simulink model "gridconnectedpvarray"  (R2023b)
settings: Solver=FixedStepDiscrete  StartTime=0.0  StopTime=2.5  RelTol=1e-3
PreLoadFcn:
  | Ts_Power=1e-6;
  | Ts_Control=100e-6;
InitFcn:
  | Ts_Power=1e-6;
  | Ts_Control=100e-6;
undefined symbols (not defined in the file): D1, Delta, DiscIntNeverNeededParam
libraries: spsSeriesRLCBranchLib x5, spsMeanLib x3, spsThreePhaseTransformerTwoWindingsLib x2, spsDistributedParametersLineLib x2, spsThreePhaseParallelRLCLoadLib x2, spsFourierLib x2, slpidlib x2, spsabctodq0Lib x2, spsVoltageMeasurementLib x2, spsThreePhaseSeriesRLCLoadLib x1, spsThreeLevelBridgeLib x1, spsThreePhaseSourceLib x1
(part 1 of 2)
settings Model: SimulationMode=accelerator  Creator=The MathWorks, Inc.  LastModifiedBy=HP
settings SolverCC: AlgebraicLoopSolver=TrustRegion
settings DataIOCC: LimitDataPoints=on  SaveFormat=Array  SignalLogging=off  DSMLogging=off  ReturnWorkspaceOutputs=off
settings OptimizationCC: ExpressionDepthLimit=2147483647  EfficientMapNaN2IntZero=off  LifeSpan=inf
settings DebuggingCC: UnderspecifiedInitializationDetection=Classic  MergeDetectMultiDrivingBlocksExec=none  SolverPrmCheckMsg=warning  FcnCallInpInsideContextMsg=warning  UnconnectedInputMsg=warning  UnconnectedOutputMsg=warning  UnconnectedLineMsg=warning  StateNameClashWarn=warning  SubsystemReferenceDiagnosticForUnitTest=warning  SFUnexpectedBacktrackingDiag=warning  SFNoUnconditionalDefaultTransitionDiag=warning  SFExecutionAtInitializationDiag=none  ArithmeticOperatorsInVariantConditions=warning
settings HardwareCC: ProdBitPerPointer=32  ProdBitPerSizeT=32  ProdBitPerPtrDiffT=32  ProdLargestAtomicFloat=None  ProdIntDivRoundTo=Undefined  ProdEndianess=Unspecified  ProdWordSize=32  ProdHWDeviceType=32-bit Generic  TargetBitPerPointer=64  TargetBitPerSizeT=64  TargetBitPerPtrDiffT=64  TargetLongLongMode=on  TargetIntDivRoundTo=Zero  TargetEndianess=LittleEndian  TargetWordSize=64  TargetHWDeviceType=MATLAB Host  ProdEqTarget=off
settings ModelReferenceCC: EnableRefExpFcnMdlSchedulingChecks=on  PropagateSignalLabelsOutOfModel=off
settings SFSimCC: SimUseLocalCustomCode=off  CustomCodeUndefinedFunction=UseInterfaceOnly
settings CodeAppCC: MaxIdLength=128
settings GRTTargetCC: TargetLangStandard=C89/C90 (ANSI)  CombineOutputUpdateFcns=off  GRTInterface=on
settings ConfigComp: CovMetricSettings=dw  CovSaveCumulativeToWorkspaceVar=on  CovSaveSingleToWorkspaceVar=on  CovExternalEMLEnable=off  CovSFcnEnable=off
settings SimscapeCC: SimscapeNormalizeSystem=off

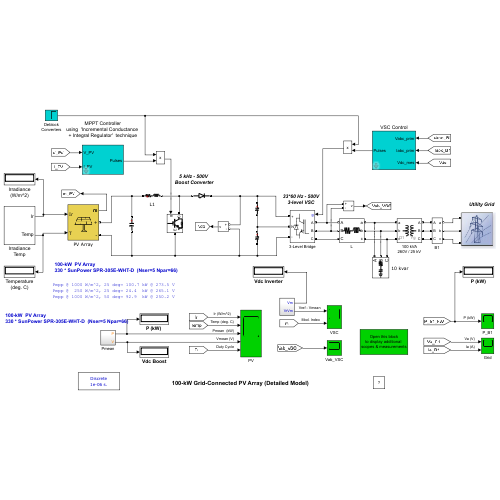
[thumbnail: Simulink's stored preview of the top-level diagram]
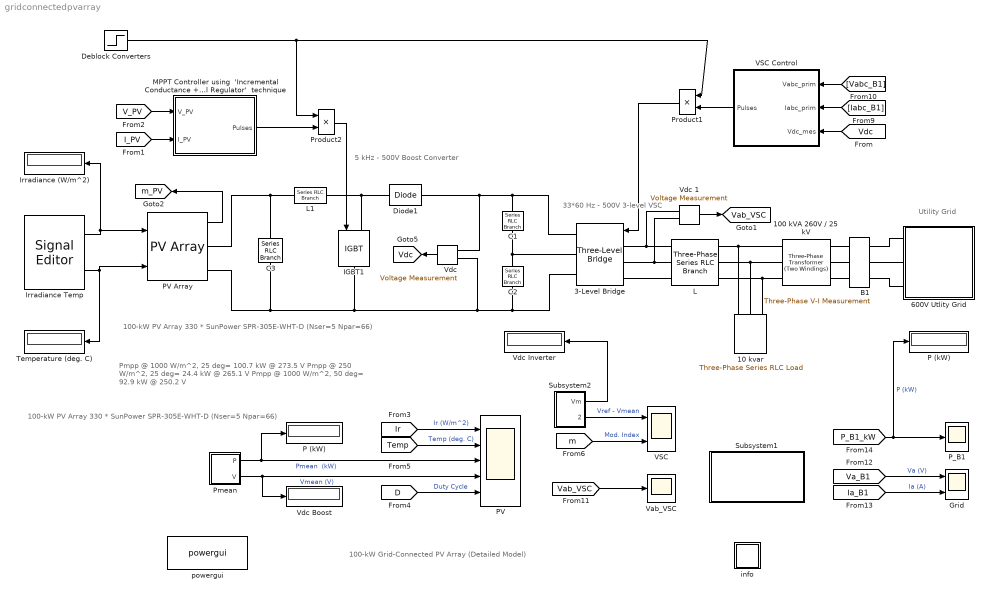
== system gridconnectedpvarray ==
  note: 5 kHz - 500V
      | Boost Converter
  note: 33*60 Hz - 500V
      | 3-level VSC
  note: 100-kW Grid-Connected PV Array (Detailed Model)
  note: Utility Grid
  note: Pmpp @ 1000 W/m^2, 25 deg= 100.7 kW @ 273.5 V
      | Pmpp @  250 W/m^2, 25 deg= 24.4  kW @ 265.1 V
      | Pmpp @ 1000 W/m^2, 50 deg= 92.9  kW @ 250.2 V
  note: 100-kW  PV Array
      | 330 * SunPower SPR-305E-WHT-D  (Nser=5 Npar=66)
  note: 100-kW  PV Array
      | 330 * SunPower SPR-305E-WHT-D  (Nser=5 Npar=66)
  10 kvar : spsThreePhaseSeriesRLCLoadLib/Three-Phase Series RLC Load  LConnTagsString=A|B|C  Configuration=Y (grounded)  NominalVoltage=240  Vabc=[1e3 1e3 1e3]  Vabcp=[1e3 1e3 1e3]  NominalFrequency=60  UnbalancedPower=off  ActivePower=10e3/100  InductivePower=0  CapacitivePower=10e3  Pabc=[10e3 9e3 11e3]  QLabc=[100 90 110]  QCabc=[100 90 110]  Pabcp=[10e3 9e3 11e3]  QLabcp=[100 90 110]  QCabcp=[100 90 110]  Measurements=None  LoadType=constant Z
  100 kVA 260V / 25 kV : spsThreePhaseTransformerTwoWindingsLib/Three-Phase Transformer (Two Windings)  Winding1Connection=Yg  Winding2Connection=Delta (D1)  CoreType=Three single-phase transformers  SetSaturation=off  Hysteresis=off  DataFile='hysteresis'  SetInitialFlux=off  Measurements=None  UNITS=pu  NominalPower=[100e3 , 60 ]  Winding1=[ 25e3 , 0.001 , 0.03 ]  Winding2=[ 260 , 0.001 , 0.03 ]  Rm=500  Lm=500  L0=0.5  Saturation=[ 0,0 ; 0.0024,1.2 ; 1.0,1.52 ]  InitialFluxes=[ 0.8 , -0.8 , 0.7 ]  BreakLoop=off  DiscreteSolver=Trapezoidal iterative  DataType=off  TransfoNumber=0
  3-Level Bridge : spsThreeLevelBridgeLib/Three-Level Bridge  Arms=3  SnubberResistance=1e6  SbubberCapacitance=inf  Device=IGBT / Diodes  Ron=0.2e-3  ForwardVoltages="[  0  0 ]"  Measurements=None
      settings: AttributesFormatString=\n
  600V Utlity Grid : Subsystem
      mask Display: image('$imagefile')
  B1 : spsThreePhaseVIMeasurementLib/Three-Phase V-I Measurement  VoltageMeasurement=phase-to-ground  SetLabelV=on  LabelV=Vabc_B1  Vpu=off  VpuLL=off  CurrentMeasurement=yes  SetLabelI=on  LabelI=Iabc_B1  Ipu=off  Pbase=100e6  Vbase=500e3  OutputType=Magnitude  PhasorSimulation=off  PSBequivalent=0
  C1 : spsSeriesRLCBranchLib/Series RLC Branch  LConnTagsString=__new0  RConnTagsString=__new0  BranchType=C  Resistance=1.0  Inductance=1.0  SetiL0=off  InitialCurrent=0  Capacitance=12000e-06  Setx0=off  InitialVoltage=0  Measurements=None
  C2 : spsSeriesRLCBranchLib/Series RLC Branch  LConnTagsString=__new0  RConnTagsString=__new0  BranchType=C  Resistance=1.0  Inductance=1.0  SetiL0=off  InitialCurrent=0  Capacitance=12000e-06  Setx0=off  InitialVoltage=0  Measurements=None
  C3 : spsSeriesRLCBranchLib/Series RLC Branch  LConnTagsString=__new0  RConnTagsString=__new0  BranchType=C  Resistance=1.0  Inductance=1.0  SetiL0=off  InitialCurrent=0  Capacitance=100e-6  Setx0=off  InitialVoltage=0  Measurements=Branch voltage
  Deblock Converters : Step  Time=0.05  SampleTime=0
  Diode1 : spsDiodeLib/Diode  Ron=1e-4  Lon=0  Vf=0  IC=0  UseSnubber=off  Rs=inf  Cs=inf  Measurements=off
  Grid : Scope  NumInputPorts=2
  IGBT1 : spsIGBTLib/IGBT  Ron=0.001  Lon=0  Vf=0  Tf=0  Tt=0  IC=0  Rs=1e5  Cs=inf  Measurements=off
  Irradiance (W/m^2) : Display
      settings: Format=bank  Decimation=1000
  Irradiance Temp : SignalEditorBlockLib/Signal Editor  FileName=PVArrayGridData.mat  ActiveScenario=Ramp_up_down_Irradiance  ActiveSignal=Temp  IsBus=off  OutputBusObjectStr=Bus: BusObject  SampleTime=0  OutputAfterFinalValue=Extrapolation  Unit=inherit  PreserveSignalName=on  ApplySigPropsToAllScenarios=on  ApplySigPropsToAllSignals=off
  L : spsThreePhaseSeriesRLCBranchLib/Three-Phase Series RLC Branch  LConnTagsString=A|B|C  RConnTagsString=A|B|C  BranchType=RL  Resistance=500e-6*377/50/2  Inductance=500e-6/2  Capacitance=inf  Measurements=None
  L1 : spsSeriesRLCBranchLib/Series RLC Branch  LConnTagsString=__new0  RConnTagsString=__new0  BranchType=RL  Resistance=0.005  Inductance=5e-3  SetiL0=off  InitialCurrent=0  Capacitance=1e-6  Setx0=off  InitialVoltage=0  Measurements=None
  "MPPT Controller using  'Incremental Conductance + Integral Regulator'  technique " : Subsystem  mask(Boost Control - MPPT){fc=5000, T_MPPT=200e-6, Dinit=0.5}
      mask prompts: fc "PWM switching frequency (Hz)"; T_MPPT "Time window used by MPPT control (s)"; Dinit "Initial value of duty cycle"
  P (kW) : Display
      settings: Format=bank  Decimation=2000
  "P (kW) " : Display
      settings: Format=bank  Decimation=2000
  PV : Scope  NumInputPorts=5
  PV Array : spsPVArrayLib/PV Array  Npar=66  Nser=5  PlotType=array @ 1000 W/m2 & specified temperatures  S_vec="[ 1000  250 ]"  Temp_C_vec="[0 25 50  ]"  ModuleName=SunPower SPR-305E-WHT-D  PlotWhenSelected=off  Pm=305.226  Ncell=96  Voc=64.2  Isc=5.96  Vm=54.7  Im=5.58  beta_Voc_pc=-0.2727  alpha_Isc_pc=0.061745  beta_Voc=-0.17507  alpha_Isc=0.00368  IL=5.9657  I0=6.3076e-12  nI=0.94489  Rsh=393.2054  Rs=0.37428  RobustModel=off  RobustCellTemperature=25  BAL=on  Tc=1e-6  Tfilter=5e-5
  P_B1 : Scope
  Pmean : Subsystem
  Product1 : Product  RndMeth=Zero
  Product2 : Product  RndMeth=Zero
  Subsystem1 : Subsystem
      mask Display: disp('Open this block\nto display additional \nscopes & measurements')
  Subsystem2 : Subsystem
  Temperature (deg. C) : Display
      settings: Format=bank  Decimation=1000
  VSC : Scope  NumInputPorts=2
  VSC Control : Subsystem  mask(VSC Main Controller){nom=[ 100e3  60 ], Vnom=[ 25e3 260 ], Vnom_dc=500, RLxfo=[0.002  0.06 ], RLchoke=[2e-3  250e-6  ], K_VDCreg=[7  800], K_Ireg=[0.3 20], Ts=Ts_Control}
      mask prompts: nom "Nominal power and frequency [ Pnom(VA)  Fnom(Hz) ]:"; Vnom "Nominal primary and secondary voltages (Vrms LL) [ Vnom_prim   Vnom_sec ]:"; Vnom_dc "Nominal DC bus voltage (V):"; RLxfo "Total transformer leakage impedance (pu/Pnom) [ Rxfo  Lxf ]"; RLchoke "Choke impedance [ R(ohm) L(H) ]"; K_VDCreg "VDC regultator gains [ Kp  Ki ]:"; K_Ireg "Current regulator gains [ Kp  Ki ]:"; Ts "Sample time"
      mask init:
      | Pnom=nom(1);
      | Fnom=nom(2);
      | Vnom_prim=Vnom(1);
      | Vnom_sec=Vnom(2);
      | Zbase=Vnom_sec^2/Pnom;
      | Rtot_pu=RLxfo(1) + RLchoke(1)/Zbase;
      | Ltot_pu=RLxfo(2) + RLchoke(2)/(Zbase/(2*pi*Fnom));
      | Kp_VDCreg=K_VDCreg(1);
      | Ki_VDCreg=K_VDCreg(2);
      | Kp_Ireg=K_Ireg(1);
      | Ki_Ireg=K_Ireg(2);
      | Vdc_ref=Vnom_dc;
      | % Used to determine initial value of Boost Control (MPPT)
      | assignin('base','Vdc_ref_Inv',Vdc_ref);
  Vab_VSC : Scope
  "Vdc " : spsVoltageMeasurementLib/Voltage Measurement  Tag=PoWeRsYsTeMmEaSuReMeNt  PhasorSimulation=off  OutputType=Magnitude  PSBequivalent=0
  Vdc 1 : spsVoltageMeasurementLib/Voltage Measurement  Tag=PoWeRsYsTeMmEaSuReMeNt  PhasorSimulation=off  OutputType=Magnitude  PSBequivalent=0
  Vdc Boost : Display
      settings: Format=bank  Decimation=2000
  Vdc Inverter : Display
      settings: Format=bank  Decimation=2000
  info : Subsystem
      settings: OpenFcn="showExample(\"simscapeelectricalsps/PVArrayGridExample\")"
      mask Display: disp('?')
  powergui : spspowerguiLib/powergui  Priority=1  SimulationMode=Discrete  SampleTime=Ts_Power  frequency=60  Iterations=50  frequencyindice=0  Pbase=100e6  ErrMax=1e-4  UnitsV=kV  UnitsW=MW  buscounter=0  FunctionMessages=off  echomessages=off  EnableUseOfTLC=off  CurrentSourceSwitches=off  DisableSnubberDevices=off  DisableRonSwitches=off  DisableVfSwitches=off  DisplayEquations=off  AutomaticDiscreteSolvers=off  SolverType=Tustin/Backward Euler (TBE)  Interpol=off  ExternalGateDelay=off  methode=off  Ts=0  x0status=blocks  SPID=off  SwTol=0  HookPort=off  NonlinearTolerance=1e-8  nMaxIteration=10  ContinueOnMaxIteration=off  RestoreLinks=warning  ResistiveCurrentMeasurement=off  Frange=[0:2:500]  Ylog=off  Xlog=on  ShowGrid=off  save=off  variable=ZData  structure=0  ZoomFFT=on  StartTime=0.0  cycles=1  DisplayStyle=1  fundamental=60  FreqAxis=off  MaxFrequency=1000  frequencyindicesteady=1  RmsSteady=1  display=off
  tag scope: Vab_VSC=global, Vdc=global, m_PV=global
  wires:
  "Vdc "/1 -> [Vdc]
  Product2/1 -> IGBT1/1
  "MPPT Controller using  'Incremental Conductance + Integral Regulator'  technique "/1(Pulses) -> Product2/2
  Deblock Converters/1 -> Product1/1, Product2/1
  [Vabc_B1] -> VSC Control/1(Vabc_prim)
  [Iabc_B1] -> VSC Control/2(Iabc_prim)
  [Vdc] -> VSC Control/3(Vdc_mes)
  VSC Control/1(Pulses) -> Product1/2
  Product1/1 -> 3-Level Bridge/1
  [I_PV] -> "MPPT Controller using  'Incremental Conductance + Integral Regulator'  technique "/2(I_PV)
  [V_PV] -> "MPPT Controller using  'Incremental Conductance + Integral Regulator'  technique "/1(V_PV)
  Pmean/1(P) -> "P (kW) "/1, PV/3  "Pmean  (kW)"
  [m] -> VSC/2  "Mod. Index"
  Vdc 1/1 -> [Vab_VSC]
  [Vab_VSC] -> Vab_VSC/1
  [Ia_B1] -> Grid/2  "Ia (A)"
  [Va_B1] -> Grid/1  "Va (V)"
  [P_B1_kW] -> P_B1/1, P (kW)/1  "P (kW)"
  Pmean/2(V) -> Vdc Boost/1, PV/4  "Vmean (V)"
  Subsystem2/2(VrVm) -> VSC/1  "Vref - Vmean"
  Subsystem2/1(Vm) -> Vdc Inverter/1
  PV Array/1 -> [m_PV]
  Irradiance Temp/1 -> PV Array/1, Irradiance (W/m^2)/1
  Irradiance Temp/2 -> PV Array/2, Temperature (deg. C)/1
  [D] -> PV/5  "Duty Cycle"
  [Temp] -> PV/2  "Temp (deg. C)"
  [Ir] -> PV/1  "Ir (W/m^2)"
  connections:
  3-Level Bridge/RConn1 -- Diode1/RConn1 -- "Vdc "/LConn1 -- C1/LConn1
  L1/RConn1 -- Diode1/LConn1 -- IGBT1/LConn1
  3-Level Bridge/RConn3 -- C2/RConn1 -- "Vdc "/LConn2 -- IGBT1/RConn1 -- PV Array/RConn2 -- C3/RConn1
  3-Level Bridge/LConn1 -- L/LConn1 -- Vdc 1/LConn1
  3-Level Bridge/LConn2 -- L/LConn2 -- Vdc 1/LConn2
  3-Level Bridge/LConn3 -- L/LConn3
  L/RConn1 -- 100 kVA 260V / 25 kV/RConn1 -- 10 kvar/LConn1
  L/RConn2 -- 100 kVA 260V / 25 kV/RConn2 -- 10 kvar/LConn2
  L/RConn3 -- 100 kVA 260V / 25 kV/RConn3 -- 10 kvar/LConn3
  B1/LConn1 -- 100 kVA 260V / 25 kV/LConn1
  B1/LConn2 -- 100 kVA 260V / 25 kV/LConn2
  B1/LConn3 -- 100 kVA 260V / 25 kV/LConn3
  C2/LConn1 -- C1/RConn1 -- 3-Level Bridge/RConn2
  C3/LConn1 -- PV Array/RConn1 -- L1/LConn1
  B1/RConn2 -- 600V Utlity Grid/LConn2
  B1/RConn1 -- 600V Utlity Grid/LConn1
  B1/RConn3 -- 600V Utlity Grid/LConn3

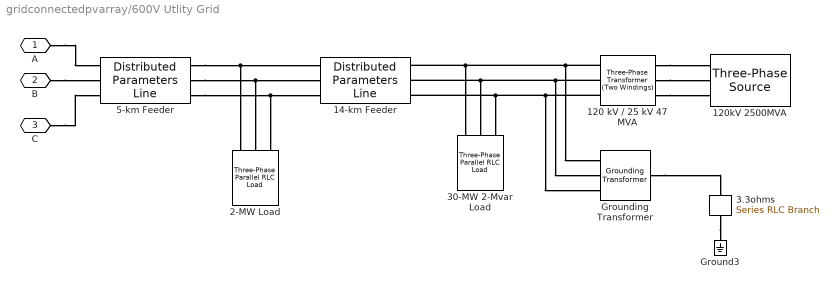
== system gridconnectedpvarray/600V Utlity Grid ==
  120 kV / 25 kV 47 MVA : spsThreePhaseTransformerTwoWindingsLib/Three-Phase Transformer (Two Windings)  Winding1Connection=Yg  Winding2Connection=Delta (D1)  CoreType=Three single-phase transformers  SetSaturation=off  Hysteresis=off  DataFile='basic_model'  SetInitialFlux=off  Measurements=None  UNITS=pu  NominalPower=[47e6 60 ]  Winding1="[ 120e3  0.08/30   0.08 ]"  Winding2="[ 25e3  0.08/30  0.08]"  Rm=500  Lm=500  L0=0.5  Saturation="[ 0,0  ;  0.005,1.2  ;  1.0,1.4 ]"  InitialFluxes=[ 0.8 , -0.8 , 0.7 ]  BreakLoop=off  DiscreteSolver=Trapezoidal iterative  DataType=off  TransfoNumber=0
  120kV 2500MVA : spsThreePhaseSourceLib/Three-Phase Source  InternalConnection=Yg  VoltagePhases=off  Voltage=120e3  PhaseAngle=0  Voltage_phases=[25e3 25e3 25e3]/sqrt(3)  PhaseAngles_phases=[0 -120 +120]  Frequency=60  NonIdealSource=on  SpecifyImpedance=on  Resistance=0.8929  Inductance=16.58e-3  ShortCircuitLevel=2500e6  BaseVoltage=120e3  XRratio=7  BusType=swing  Pref=0  Qref=0  Prefabc=[10e3, 10e3, 10e3]  Qrefabc=[0, 0, 0]  Qmin=-inf  Qmax=inf
  14-km Feeder : spsDistributedParametersLineLib/Distributed Parameters Line  Phases=3  Length=14  Frequency=60  Resistance=[0.1153 0.413]  Inductance=[1.05e-3 3.32e-3]  Capacitance=[11.33e-009 5.01e-009]  x1=[-5.8e-05 6.66844526107812e-10 0 0;-5.7e-05 6.67988838949903e-10 0 0;-5.6e-05 6.69133056855883e-10 0 0;-5.5e-05 6.70277179663133e-10 0 0;-5.4e-05 6.71421207209047e-10 0 0;-5.3e-05 6.72565139331033e-10 0 0;-5.2e-05 6.73708975866514e-10 0 0;-5.1e-05 6.74852716652925e-10 0 0;-5e-05 6.75996361527714e-10 0 0;-4.9e-05 6.77139910328345e-10 -3790.73535190058 -24061.4134200257;-4.8e-05 6.78283362892292e-10 -3781.66414358518 -24062.8407837201;-4.7e-05 6.79426719057047e-10 -3772.59239781097 -24064.2647275482;-4.6e-05 6.80569978660113e-10 -3763.52011586725 -24065.6852513076;-4.5e-05 6.81713141539008e-10 -3754.44729904339 -24067.1023547964;-4.4e-05 6.82856207531261e-10 -3745.37394862884 -24068.5160378133;-4.3e-05 6.83999176474418e-10 -3736.30006591311 -24069.9263001572;-4.2e-05 6.85142048206038e-10 -3727.22565218583 -24071.3331416278;-4.1e-05 6.86284822563693e-10 -3718.15070873665 -24072.7365620252;-4e-05 6.8742749938497e-10 -3709.07523685534 -24074.1365611498;-3.9e-05 6.88570078507468e-10 -3699.99923783172 -24075.5331388027;-3.8e-05 6.89712559768802e-10 -3690.92271295569 -24076.9262947854;-3.7e-05 6.90854943006599e-10 -3681.84566351723 -24078.3160289;-3.6e-05 6.91997228058502e-10 -3672.76809080639 -24079.7023409488;-3.5e-05 6.93139414762165e-10 -3663.6899961133 -24081.0852307349;-3.4e-05 6.9428150295526e-10 -3654.61138072814 -24082.4646980618;-3.3e-05 6.9542349247547e-10 -3645.53224594121 -24083.8407427334;-3.2e-05 6.96565383160492e-10 -3636.45259304285 -24085.213364554;-3.1e-05 6.97707174848038e-10 -3627.37242332347 -24086.5825633288;-3e-05 6.98848867375835e-10 -3618.29173807357 -24087.9483388629;-2.9e-05 6.99990460581623e-10 -3609.21053858373 -24089.3106909624;-2.8e-05 7.01131954303155e-10 -3600.12882614457 -24090.6696194337;-2.7e-05 7.022733483782e-10 -3591.04660204683 -24092.0251240835;-2.6e-05 7.0341464264454e-10 -3581.96386758127 -24093.3772047192;-2.5e-05 7.04555836939972e-10 -3572.88062403876 -24094.7258611487;-2.4e-05 7.05696931102307e-10 -3563.79687271023 -24096.0710931803;-2.3e-05 7.0683792496937e-10 -3554.71261488669 -24097.4129006229;-2.2e-05 7.07978818378999e-10 -3545.62785185921 -24098.7512832856;-2.1e-05 7.0911961116905e-10 -3536.54258491894 -24100.0862409784;-2e-05 7.1026030317739e-10 -3527.4568153571 -24101.4177735114;-1.9e-05 7.114008942419e-10 -3518.37054446498 -24102.7458806954;-1.8e-05 7.12541384200478e-10 -3509.28377353393 -24104.0705623418;-1.7e-05 7.13681772891034e-10 -3500.1965038554 -24105.3918182621;-1.6e-05 7.14822060151494e-10 -3491.10873672089 -24106.7096482687;-1.5e-05 7.15962245819797e-10 -3482.02047342196 -24108.0240521742;-1.4e-05 7.17102329733899e-10 -3472.93171525028 -24109.3350297919;-1.3e-05 7.18242311731766e-10 -3463.84246349754 -24110.6425809353;-1.2e-05 7.19382191651383e-10 -3454.75271945554 -24111.9467054188;-1.1e-05 7.20521969330747e-10 -3445.66248441613 -24113.2474030568;-1e-05 7.21661644607871e-10 -3436.57175967124 -24114.5446736647;-9e-06 7.2280121732078e-10 -3427.48054651286 -24115.838517058;-8e-06 7.23940687307517e-10 -3418.38884623305 -24117.1289330527;-7e-06 7.25080054406137e-10 -3409.29666012396 -24118.4159214656;-6e-06 7.26219318454711e-10 -3400.20398947777 -24119.6994821138;-5e-06 7.27358479291324e-10 -3391.11083558677 -24120.9796148147;-4e-06 7.28497536754075e-10 -3382.01719974329 -24122.2563193865;-3e-06 7.2963649068108e-10 -3372.92308323975 -24123.5295956477;-2e-06 7.30775340910467e-10 -3363.82848736861 -24124.7994434173;-1e-06 7.31914087280381e-10 -3354.73341342242 -24126.0658625149]  x2=[-5.8e-05 8.33047014327362e-10 0 0;-5.7e-05 8.34243099749187e-10 0 0;-5.6e-05 8.35439066606464e-10 0 0;-5.5e-05 8.36634914729217e-10 0 0;-5.4e-05 8.37830643947491e-10 0 0;-5.3e-05 8.39026254091345e-10 0 0;-5.2e-05 8.40221744990856e-10 0 0;-5.1e-05 8.4141711647612e-10 0 0;-5e-05 8.42612368377246e-10 0 0;-4.9e-05 8.43807500524362e-10 -3379.3924259141 -24244.0512732158;-4.8e-05 8.45002512747615e-10 -3370.2523939823 -24245.3235513057;-4.7e-05 8.46197404877165e-10 -3361.11188306246 -24246.5923835944;-4.6e-05 8.47392176743193e-10 -3351.97089445368 -24247.8577699016;-4.5e-05 8.48586828175894e-10 -3342.82942945507 -24249.1197100474;-4.4e-05 8.49781359005482e-10 -3333.68748936585 -24250.3782038526;-4.3e-05 8.50975769062187e-10 -3324.54507548529 -24251.6332511381;-4.2e-05 8.52170058176258e-10 -3315.40218911273 -24252.8848517258;-4.1e-05 8.53364226177958e-10 -3306.25883154759 -24254.1330054376;-4e-05 8.5455827289757e-10 -3297.11500408932 -24255.3777120962;-3.9e-05 8.55752198165393e-10 -3287.97070803749 -24256.6189715247;-3.8e-05 8.56946001811744e-10 -3278.82594469169 -24257.8567835466;-3.7e-05 8.58139683666958e-10 -3269.6807153516 -24259.0911479861;-3.6e-05 8.59333243561384e-10 -3260.53502131696 -24260.3220646678;-3.5e-05 8.60526681325391e-10 -3251.38886388758 -24261.5495334167;-3.4e-05 8.61719996789366e-10 -3242.24224436333 -24262.7735540582;-3.3e-05 8.62913189783712e-10 -3233.09516404414 -24263.9941264186;-3.2e-05 8.64106260138849e-10 -3223.94762423004 -24265.2112503243;-3.1e-05 8.65299207685215e-10 -3214.79962622107 -24266.4249256023;-3e-05 8.66492032253267e-10 -3205.65117131739 -24267.6351520801;-2.9e-05 8.67684733673476e-10 -3196.50226081918 -24268.8419295858;-2.8e-05 8.68877311776334e-10 -3187.35289602671 -24270.0452579477;-2.7e-05 8.70069766392348e-10 -3178.20307824031 -24271.245136995;-2.6e-05 8.71262097352045e-10 -3169.05280876038 -24272.4415665571;-2.5e-05 8.72454304485967e-10 -3159.90208888736 -24273.6345464639;-2.4e-05 8.73646387624675e-10 -3150.75091992179 -24274.8240765459;-2.3e-05 8.74838346598747e-10 -3141.59930316424 -24276.010156634;-2.2e-05 8.7603018123878e-10 -3132.44723991538 -24277.1927865597;-2.1e-05 8.77221891375388e-10 -3123.29473147589 -24278.3719661549;-2e-05 8.78413476839201e-10 -3114.14177914658 -24279.547695252;-1.9e-05 8.79604937460869e-10 -3104.98838422826 -24280.7199736838;-1.8e-05 8.80796273071058e-10 -3095.83454802185 -24281.8888012839;-1.7e-05 8.81987483500454e-10 -3086.68027182831 -24283.054177886;-1.6e-05 8.83178568579759e-10 -3077.52555694867 -24284.2161033246;-1.5e-05 8.84369528139693e-10 -3068.370404684 -24285.3745774345;-1.4e-05 8.85560362010994e-10 -3059.21481633548 -24286.529600051;-1.3e-05 8.86751070024418e-10 -3050.0587932043 -24287.6811710101;-1.2e-05 8.87941652010739e-10 -3040.90233659175 -24288.829290148;-1.1e-05 8.89132107800748e-10 -3031.74544779915 -24289.9739573016;-1e-05 8.90322437225256e-10 -3022.58812812792 -24291.1151723082;-9e-06 8.9151264011509e-10 -3013.4303788795 -24292.2529350056;-8e-06 8.92702716301095e-10 -3004.27220135543 -24293.3872452321;-7e-06 8.93892665614136e-10 -2995.11359685727 -24294.5181028264;-6e-06 8.95082487885093e-10 -2985.95456668667 -24295.645507628;-5e-06 8.96272182944868e-10 -2976.79511214534 -24296.7694594765;-4e-06 8.97461750624376e-10 -2967.63523453504 -24297.8899582121;-3e-06 8.98651190754555e-10 -2958.47493515758 -24299.0070036758;-2e-06 8.99840503166358e-10 -2949.31421531486 -24300.1205957086;-1e-06 9.01029687690758e-10 -2940.15307630881 -24301.2307341524]  x3=[-5.8e-05 -3.7534649390882e-12 0 0;-5.7e-05 -3.74760398121956e-12 0 0;-5.6e-05 -3.74174249073282e-12 0 0;-5.5e-05 -3.73588046846102e-12 0 0;-5.4e-05 -3.7300179152373e-12 0 0;-5.3e-05 -3.72415483189484e-12 0 0;-5.2e-05 -3.71829121926693e-12 0 0;-5.1e-05 -3.7124270781869e-12 0 0;-5e-05 -3.7065624094882e-12 0 0;-4.9e-05 -3.70069721400432e-12 -23.5442847382658 -155.68147777383;-4.8e-05 -3.69483149256883e-12 -23.4855925321471 -155.690342696951;-4.7e-05 -3.68896524601538e-12 -23.426896988202 -155.699185493002;-4.6e-05 -3.68309847517771e-12 -23.3681981147723 -155.708006160726;-4.5e-05 -3.6772311808896e-12 -23.3094959202006 -155.716804698871;-4.4e-05 -3.67136336398493e-12 -23.2507904128296 -155.725581106184;-4.3e-05 -3.66549502529765e-12 -23.1920816010027 -155.73433538142;-4.2e-05 -3.65962616566178e-12 -23.1333694930639 -155.743067523333;-4.1e-05 -3.65375678591142e-12 -23.0746540973573 -155.751777530683;-4e-05 -3.64788688688073e-12 -23.0159354222278 -155.760465402232;-3.9e-05 -3.64201646940396e-12 -22.9572134760206 -155.769131136745;-3.8e-05 -3.63614553431543e-12 -22.8984882670813 -155.777774732991;-3.7e-05 -3.63027408244952e-12 -22.8397598037562 -155.78639618974;-3.6e-05 -3.62440211464071e-12 -22.7810280943919 -155.794995505769;-3.5e-05 -3.61852963172352e-12 -22.7222931473354 -155.803572679854;-3.4e-05 -3.61265663453258e-12 -22.6635549709343 -155.812127710777;-3.3e-05 -3.60678312390256e-12 -22.6048135735366 -155.820660597322;-3.2e-05 -3.60090910066822e-12 -22.5460689634907 -155.829171338275;-3.1e-05 -3.59503456566439e-12 -22.4873211491457 -155.837659932428;-3e-05 -3.58915951972597e-12 -22.4285701388508 -155.846126378575;-2.9e-05 -3.58328396368794e-12 -22.3698159409559 -155.854570675511;-2.8e-05 -3.57740789838535e-12 -22.3110585638113 -155.862992822037;-2.7e-05 -3.57153132465331e-12 -22.2522980157677 -155.871392816955;-2.6e-05 -3.56565424332702e-12 -22.1935343051762 -155.879770659072;-2.5e-05 -3.55977665524175e-12 -22.1347674403886 -155.888126347198;-2.4e-05 -3.55389856123282e-12 -22.0759974297569 -155.896459880144;-2.3e-05 -3.54801996213564e-12 -22.0172242816336 -155.904771256727;-2.2e-05 -3.5421408587857e-12 -21.9584480043718 -155.913060475764;-2.1e-05 -3.53626125201856e-12 -21.8996686063247 -155.921327536079;-2e-05 -3.53038114266982e-12 -21.8408860958464 -155.929572436495;-1.9e-05 -3.52450053157519e-12 -21.782100481291 -155.937795175842;-1.8e-05 -3.51861941957043e-12 -21.7233117710134 -155.945995752951;-1.7e-05 -3.51273780749138e-12 -21.6645199733688 -155.954174166655;-1.6e-05 -3.50685569617395e-12 -21.6057250967126 -155.962330415794;-1.5e-05 -3.50097308645411e-12 -21.5469271494011 -155.970464499207;-1.4e-05 -3.49508997916792e-12 -21.4881261397908 -155.978576415739;-1.3e-05 -3.4892063751515e-12 -21.4293220762384 -155.986666164236;-1.2e-05 -3.48332227524104e-12 -21.3705149671015 -155.994733743549;-1.1e-05 -3.4774376802728e-12 -21.3117048207378 -156.002779152532;-1e-05 -3.47155259108311e-12 -21.2528916455056 -156.010802390041;-9e-06 -3.46566700850838e-12 -21.1940754497635 -156.018803454935;-8e-06 -3.45978093338507e-12 -21.1352562418706 -156.026782346078;-7e-06 -3.45389436654974e-12 -21.0764340301865 -156.034739062336;-6e-06 -3.44800730883899e-12 -21.017608823071 -156.042673602577;-5e-06 -3.4421197610895e-12 -20.9587806288846 -156.050585965674;-4e-06 -3.43623172413803e-12 -20.8999494559881 -156.058476150503;-3e-06 -3.4303431988214e-12 -20.8411153127426 -156.066344155942;-2e-06 -3.42445418597649e-12 -20.7822782075098 -156.074189980873;-1e-06 -3.41856468644028e-12 -20.7234381486519 -156.082013624181]  x4=[-5.8e-05 5.86381987524126e-12 0 0;-5.7e-05 5.86113014706762e-12 0 0;-5.6e-05 5.85843958589666e-12 0 0;-5.5e-05 5.85574819211079e-12 0 0;-5.4e-05 5.8530559660925e-12 0 0;-5.3e-05 5.85036290822443e-12 0 0;-5.2e-05 5.84766901888932e-12 0 0;-5.1e-05 5.84497429847002e-12 0 0;-5e-05 5.84227874734953e-12 0 0;-4.9e-05 5.83958236591093e-12 -1.35581366009685 -2.15298522697963;-4.8e-05 5.83688515453745e-12 -1.35500190746171 -2.15349620368202;-4.7e-05 5.83418711361241e-12 -1.35418996225058 -2.15400687432457;-4.6e-05 5.83148824351927e-12 -1.35337782457886 -2.15451723883471;-4.5e-05 5.8287885446416e-12 -1.35256549456196 -2.1550272971399;-4.4e-05 5.82608801736309e-12 -1.35175297231535 -2.15553704916764;-4.3e-05 5.82338666206754e-12 -1.35094025795449 -2.15604649484551;-4.2e-05 5.82068447913887e-12 -1.35012735159489 -2.15655563410108;-4.1e-05 5.81798146896113e-12 -1.34931425335208 -2.157064466862;-4e-05 5.81527763191847e-12 -1.34850096334163 -2.15757299305595;-3.9e-05 5.81257296839516e-12 -1.34768748167912 -2.15808121261067;-3.8e-05 5.80986747877561e-12 -1.34687380848016 -2.15858912545391;-3.7e-05 5.80716116344432e-12 -1.34605994386039 -2.1590967315135;-3.6e-05 5.80445402278592e-12 -1.34524588793549 -2.1596040307173;-3.5e-05 5.80174605718515e-12 -1.34443164082114 -2.16011102299319;-3.4e-05 5.79903726702688e-12 -1.34361720263308 -2.16061770826914;-3.3e-05 5.79632765269608e-12 -1.34280257348704 -2.16112408647313;-3.2e-05 5.79361721457786e-12 -1.34198775349882 -2.16163015753318;-3.1e-05 5.79090595305742e-12 -1.3411727427842 -2.16213592137738;-3e-05 5.7881938685201e-12 -1.34035754145903 -2.16264137793385;-2.9e-05 5.78548096135135e-12 -1.33954214963916 -2.16314652713075;-2.8e-05 5.78276723193672e-12 -1.33872656744047 -2.16365136889629;-2.7e-05 5.78005268066191e-12 -1.33791079497889 -2.16415590315871;-2.6e-05 5.7773373079127e-12 -1.33709483237034 -2.16466012984631;-2.5e-05 5.77462111407503e-12 -1.3362786797308 -2.16516404888744;-2.4e-05 5.7719040995349e-12 -1.33546233717626 -2.16566766021046;-2.3e-05 5.76918626467848e-12 -1.33464580482273 -2.16617096374382;-2.2e-05 5.76646760989203e-12 -1.33382908278627 -2.16667395941597;-2.1e-05 5.76374813556193e-12 -1.33301217118295 -2.16717664715543;-2e-05 5.76102784207467e-12 -1.33219507012888 -2.16767902689076;-1.9e-05 5.75830672981688e-12 -1.33137777974017 -2.16818109855055;-1.8e-05 5.75558479917529e-12 -1.33056030013299 -2.16868286206346;-1.7e-05 5.75286205053673e-12 -1.32974263142352 -2.16918431735816;-1.6e-05 5.75013848428818e-12 -1.32892477372796 -2.1696854643634;-1.5e-05 5.74741410081672e-12 -1.32810672716256 -2.17018630300795;-1.4e-05 5.74468890050953e-12 -1.32728849184357 -2.17068683322062;-1.3e-05 5.74196288375393e-12 -1.32647006788728 -2.17118705493028;-1.2e-05 5.73923605093735e-12 -1.32565145541002 -2.17168696806585;-1.1e-05 5.73650840244734e-12 -1.32483265452812 -2.17218657255626;-1e-05 5.73377993867154e-12 -1.32401366535795 -2.17268586833052;-9e-06 5.73105065999775e-12 -1.32319448801592 -2.17318485531766;-8e-06 5.72832056681384e-12 -1.32237512261844 -2.17368353344676;-7e-06 5.72558965950783e-12 -1.32155556928196 -2.17418190264696;-6e-06 5.72285793846784e-12 -1.32073582812296 -2.17467996284743;-5e-06 5.7201254040821e-12 -1.31991589925795 -2.17517771397737;-4e-06 5.71739205673898e-12 -1.31909578280345 -2.17567515596605;-3e-06 5.71465789682694e-12 -1.31827547887602 -2.17617228874276;-2e-06 5.71192292473456e-12 -1.31745498759225 -2.17666911223687;-1e-06 5.70918714085056e-12 -1.31663430906874 -2.17716562637775]  x5=5.70973484498186e-05  V1=[0 0 0 2.868e-09 2.436e+04 2.436e+04;0 0 0 377 377 377;1.571 1.571 1.571 -0.5389 -0.156 -1.727]  V2=[0 0 0 2.996e-09 2.448e+04 2.448e+04;0 0 0 377 377 377;1.571 1.571 1.571 -0.5232 -0.1382 -1.709]  I1=[0 0 0 1.022e-11 157.5 157.5;0 0 0 377 377 377;1.571 1.571 1.571 -1.198 -0.1498 -1.721]  I2=[0 0 0 6.231e-12 2.544 2.544;0 0 0 377 377 377;1.571 1.571 1.571 1.184 -0.5617 -2.133]  nHarmo=2  Measurements=None  Decoupling=off  VsMag0=0  VrMag0=0  VsAngle0=0  VrAngle0=0  IsMag0=0  IrMag0=0  IsAngle0=0  IrAngle0=0
  2-MW Load : spsThreePhaseParallelRLCLoadLib/Three-Phase Parallel RLC Load  LConnTagsString=A|B|C  Configuration=Y (grounded)  NominalVoltage=25e3  Vabc=[1e3 1e3 1e3]  Vabcp=[1e3 1e3 1e3]  NominalFrequency=60  UnbalancedPower=off  ActivePower=2e6  InductivePower=0  CapacitivePower=0  Pabc=[10e3 9e3 11e3]  QLabc=[100 90 110]  QCabc=[100 90 110]  Pabcp=[10e3 9e3 11e3]  QLabcp=[100 90 110]  QCabcp=[100 90 110]  Measurements=None  LoadType=constant Z
  "3.3ohms " : spsSeriesRLCBranchLib/Series RLC Branch  LConnTagsString=__new0  RConnTagsString=__new0  BranchType=R  Resistance=3.3  Inductance=[]  SetiL0=off  InitialCurrent=0  Capacitance=[]  Setx0=off  InitialVoltage=0  Measurements=None
  30-MW 2-Mvar Load : spsThreePhaseParallelRLCLoadLib/Three-Phase Parallel RLC Load  LConnTagsString=A|B|C  Configuration=Y (grounded)  NominalVoltage=25e3  Vabc=[1e3 1e3 1e3]  Vabcp=[1e3 1e3 1e3]  NominalFrequency=60  UnbalancedPower=off  ActivePower=30e6  InductivePower=2e6  CapacitivePower=0  Pabc=[10e3 9e3 11e3]  QLabc=[100 90 110]  QCabc=[100 90 110]  Pabcp=[10e3 9e3 11e3]  QLabcp=[100 90 110]  QCabcp=[100 90 110]  Measurements=None  LoadType=constant Z
  5-km Feeder : spsDistributedParametersLineLib/Distributed Parameters Line  Phases=3  Length=5  Frequency=60  Resistance=[0.1153 0.413]  Inductance=[1.05e-3 3.32e-3]  Capacitance=[11.33e-009 5.01e-009]  x1=[-2.1e-05 7.25963417547269e-10 -3537.17773129719 -24101.4118174696;-2e-05 7.27081614129065e-10 -3528.09146195966 -24102.743589353;-1.9e-05 7.28199707376349e-10 -3519.00469120165 -24104.071935699;-1.8e-05 7.29317697130214e-10 -3509.9174203146 -24105.3968563187;-1.7e-05 7.30435583231769e-10 -3500.82965059 -24106.718351024;-1.6e-05 7.31553365522139e-10 -3491.74138331944 -24108.036419627;-1.5e-05 7.3267104384246e-10 -3482.65261979455 -24109.3510619404;-1.4e-05 7.33788618033886e-10 -3473.56336130706 -24110.6622777773;-1.3e-05 7.34906087937584e-10 -3464.47360914875 -24111.9700669514;-1.2e-05 7.36023453394738e-10 -3455.38336461147 -24113.2744292768;-1.1e-05 7.37140714246545e-10 -3446.29262898716 -24114.5753645682;-1e-05 7.38257870334216e-10 -3437.2014035678 -24115.8728726406;-9e-06 7.3937492149898e-10 -3428.10968964547 -24117.1669533096;-8e-06 7.40491867582078e-10 -3419.0174885123 -24118.4576063913;-7e-06 7.41608708424768e-10 -3409.9248014605 -24119.7448317024;-6e-06 7.42725443868321e-10 -3400.83162978233 -24121.0286290598;-5e-06 7.43842073754024e-10 -3391.73797477015 -24122.3089982811;-4e-06 7.4495859792318e-10 -3382.64383771636 -24123.5859391843;-3e-06 7.46075016217105e-10 -3373.54921991344 -24124.8594515879;-2e-06 7.47191328477132e-10 -3364.45412265394 -24126.129535311;-1e-06 7.48307534544607e-10 -3355.35854723048 -24127.396190173]  x2=[-2.1e-05 7.0911961116905e-10 -3536.54258491894 -24100.0862409784;-2e-05 7.1026030317739e-10 -3527.4568153571 -24101.4177735114;-1.9e-05 7.114008942419e-10 -3518.37054446498 -24102.7458806954;-1.8e-05 7.12541384200478e-10 -3509.28377353393 -24104.0705623418;-1.7e-05 7.13681772891034e-10 -3500.1965038554 -24105.3918182621;-1.6e-05 7.14822060151494e-10 -3491.10873672089 -24106.7096482687;-1.5e-05 7.15962245819797e-10 -3482.02047342196 -24108.0240521742;-1.4e-05 7.17102329733899e-10 -3472.93171525028 -24109.3350297919;-1.3e-05 7.18242311731766e-10 -3463.84246349754 -24110.6425809353;-1.2e-05 7.19382191651383e-10 -3454.75271945554 -24111.9467054188;-1.1e-05 7.20521969330747e-10 -3445.66248441613 -24113.2474030568;-1e-05 7.21661644607871e-10 -3436.57175967124 -24114.5446736647;-9e-06 7.2280121732078e-10 -3427.48054651286 -24115.838517058;-8e-06 7.23940687307517e-10 -3418.38884623305 -24117.1289330527;-7e-06 7.25080054406137e-10 -3409.29666012396 -24118.4159214656;-6e-06 7.26219318454711e-10 -3400.20398947777 -24119.6994821138;-5e-06 7.27358479291324e-10 -3391.11083558677 -24120.9796148147;-4e-06 7.28497536754075e-10 -3382.01719974329 -24122.2563193865;-3e-06 7.2963649068108e-10 -3372.92308323975 -24123.5295956477;-2e-06 7.30775340910467e-10 -3363.82848736861 -24124.7994434173;-1e-06 7.31914087280381e-10 -3354.73341342242 -24126.0658625149]  x3=[-2.1e-05 -1.01310369307852e-11 -11.1569792961419 -79.1361755515047;-2e-05 -1.01294879791258e-11 -11.1271448686913 -79.1403760100006;-1.9e-05 -1.01279375878404e-11 -11.0973088598252 -79.144565220884;-1.8e-05 -1.01263857571491e-11 -11.0674712737841 -79.1487431835596;-1.7e-05 -1.01248324872725e-11 -11.0376321148085 -79.1529098974337;-1.6e-05 -1.01232777784315e-11 -11.0077913871392 -79.1570653619141;-1.5e-05 -1.01217216308469e-11 -10.9779490950172 -79.1612095764101;-1.4e-05 -1.012016404474e-11 -10.9481052426839 -79.1653425403328;-1.3e-05 -1.0118605020332e-11 -10.9182598343806 -79.1694642530948;-1.2e-05 -1.01170445578447e-11 -10.8884128743491 -79.1735747141104;-1.1e-05 -1.01154826574996e-11 -10.8585643668313 -79.1776739227952;-1e-05 -1.01139193195189e-11 -10.8287143160694 -79.1817618785668;-9e-06 -1.01123545441247e-11 -10.7988627263057 -79.1858385808442;-8e-06 -1.01107883315394e-11 -10.7690096017827 -79.1899040290479;-7e-06 -1.01092206819855e-11 -10.7391549467433 -79.1939582226002;-6e-06 -1.0107651595686e-11 -10.7092987654305 -79.1980011609248;-5e-06 -1.01060810728637e-11 -10.6794410620874 -79.2020328434473;-4e-06 -1.0104509113742e-11 -10.6495818409577 -79.2060532695945;-3e-06 -1.01029357185441e-11 -10.6197211062848 -79.2100624387952;-2e-06 -1.01013608874938e-11 -10.5898588623128 -79.2140603504794;-1e-06 -1.00997846208148e-11 -10.5599951132856 -79.2180470040791]  x4=[-2.1e-05 1.05230369852105e-11 -12.5606324026043 -78.9000787577079;-2e-05 1.05244491397287e-11 -12.5308868818007 -78.904808397723;-1.9e-05 1.0525859798488e-11 -12.5011395800787 -78.9095268236051;-1.8e-05 1.05272689612879e-11 -12.4713905016659 -78.9142340346836;-1.7e-05 1.0528676627928e-11 -12.4416396507904 -78.9189300302896;-1.6e-05 1.05300827982085e-11 -12.4118870316804 -78.9236148097556;-1.5e-05 1.05314874719293e-11 -12.3821326485644 -78.9282883724158;-1.4e-05 1.05328906488908e-11 -12.3523765056713 -78.9329507176059;-1.3e-05 1.05342923288937e-11 -12.32261860723 -78.9376018446634;-1.2e-05 1.05356925117388e-11 -12.2928589574698 -78.9422417529273;-1.1e-05 1.05370911972269e-11 -12.2630975606201 -78.9468704417381;-1e-05 1.05384883851594e-11 -12.2333344209108 -78.9514879104379;-9e-06 1.05398840753377e-11 -12.2035695425719 -78.9560941583705;-8e-06 1.05412782675634e-11 -12.1738029298336 -78.9606891848814;-7e-06 1.05426709616384e-11 -12.1440345869264 -78.9652729893173;-6e-06 1.05440621573647e-11 -12.114264518081 -78.9698455710268;-5e-06 1.05454518545446e-11 -12.0844927275285 -78.9744069293602;-4e-06 1.05468400529806e-11 -12.0547192195 -78.978957063669;-3e-06 1.05482267524755e-11 -12.0249439982272 -78.9834959733067;-2e-06 1.0549611952832e-11 -11.9951670679416 -78.9880236576282;-1e-06 1.05509956538535e-11 -11.9653884328752 -78.9925401159899]  x5=2.03919101606495e-05  V1=[0 0 0 2.827e-09 2.436e+04 2.436e+04;0 0 0 377 377 377;1.571 1.571 1.571 -0.5179 -0.1443 -1.715]  V2=[0 0 0 2.868e-09 2.436e+04 2.436e+04;0 0 0 377 377 377;1.571 1.571 1.571 -0.5251 -0.1443 -1.715]  I1=[0 0 0 7.018e-12 79.92 79.92;0 0 0 377 377 377;1.571 1.571 1.571 -1.622 -0.1386 -1.709]  I2=[0 0 0 7.946e-12 79.89 79.89;0 0 0 377 377 377;1.571 1.571 1.571 0.3547 -0.1565 -1.727]  nHarmo=2  Measurements=None  Decoupling=off  VsMag0=0  VrMag0=0  VsAngle0=0  VrAngle0=0  IsMag0=0  IrMag0=0  IsAngle0=0  IrAngle0=0
  Ground3 : spsGroundLib/Ground  LConnTagsString=a
  "Grounding Transformer " : spsGroundingTransformerLib/Grounding Transformer   UNITS=pu  NominalPower="[100e6   60]"  NominalVoltage=25e3  ZeroSequenceImpedance_pu=[0.025 0.75]  MagnetizationBranch_pu=[500 500]  ZeroSequenceImpedance_SI=[0.052083 589.05]  MagnetizationBranch_SI=[1041.7 3.927e+005]  Measurements=None
  A : PMIOPort  Side=Left
  B : PMIOPort  Port=2  Side=Left
  C : PMIOPort  Port=3  Side=Left
  connections:
  "3.3ohms "/RConn1 -- Ground3/LConn1
  120 kV / 25 kV 47 MVA/LConn1 -- 120kV 2500MVA/RConn1
  120 kV / 25 kV 47 MVA/LConn2 -- 120kV 2500MVA/RConn2
  120 kV / 25 kV 47 MVA/LConn3 -- 120kV 2500MVA/RConn3
  120 kV / 25 kV 47 MVA/RConn1 -- "Grounding Transformer "/LConn1 -- 14-km Feeder/RConn1 -- 30-MW 2-Mvar Load/LConn1
  120 kV / 25 kV 47 MVA/RConn2 -- "Grounding Transformer "/LConn2 -- 14-km Feeder/RConn2 -- 30-MW 2-Mvar Load/LConn2
  120 kV / 25 kV 47 MVA/RConn3 -- "Grounding Transformer "/LConn3 -- 14-km Feeder/RConn3 -- 30-MW 2-Mvar Load/LConn3
  5-km Feeder/RConn1 -- 14-km Feeder/LConn1 -- 2-MW Load/LConn1
  5-km Feeder/RConn2 -- 14-km Feeder/LConn2 -- 2-MW Load/LConn2
  5-km Feeder/RConn3 -- 14-km Feeder/LConn3 -- 2-MW Load/LConn3
  A/RConn1 -- 5-km Feeder/LConn1
  B/RConn1 -- 5-km Feeder/LConn2
  C/RConn1 -- 5-km Feeder/LConn3
  "Grounding Transformer "/RConn1 -- "3.3ohms "/LConn1

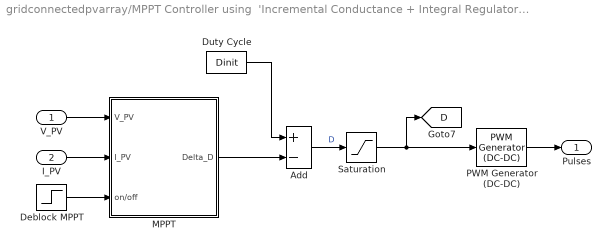
== system gridconnectedpvarray/MPPT Controller using  'Incremental Conductance + Integral Regulator'  technique  ==
  V_PV : Inport
  I_PV : Inport  Port=2
  Add : Sum  Inputs=+-
  Deblock MPPT : Step  Time=0.4  SampleTime=0
  Duty Cycle : Constant  Value=Dinit
  MPPT : Subsystem
  PWM Generator (DC-DC) : spsPWMGeneratorDCDCLib/PWM Generator (DC-DC)  Fsw=fc  Ts=Ts_Power
  Saturation : Saturate  UpperLimit=1  LowerLimit=0
  Pulses : Outport  VectorParamsAs1DForOutWhenUnconnected=off
  tag scope: D=global
  wires:
  V_PV/1 -> MPPT/1(V_PV)
  I_PV/1 -> MPPT/2(I_PV)
  PWM Generator (DC-DC)/1 -> Pulses/1
  Deblock MPPT/1 -> MPPT/3(on/off)
  Saturation/1 -> PWM Generator (DC-DC)/1, [D]
  Add/1 -> Saturation/1  "D"
  MPPT/1(Delta_D) -> Add/2
  Duty Cycle/1 -> Add/1

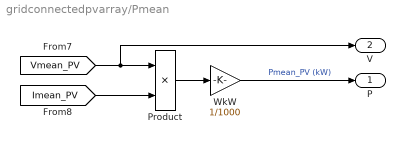
== system gridconnectedpvarray/Pmean ==
  Product : Product  RndMeth=Zero
  WkW : Gain  Gain=1/1000
  P : Outport  VectorParamsAs1DForOutWhenUnconnected=off
  V : Outport  Port=2  VectorParamsAs1DForOutWhenUnconnected=off
  wires:
  [Vmean_PV] -> Product/1, V/1
  Product/1 -> WkW/1
  [Imean_PV] -> Product/2
  WkW/1 -> P/1  "Pmean_PV (kW)"

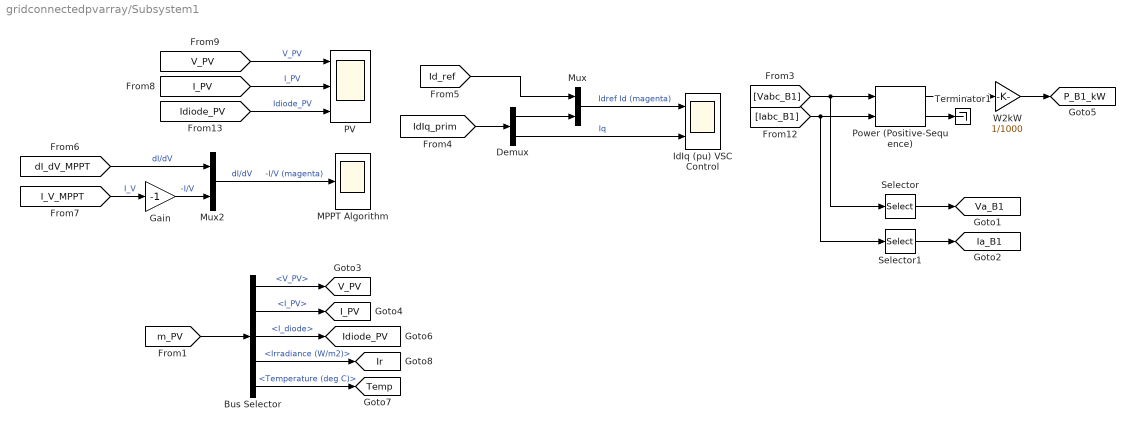
== system gridconnectedpvarray/Subsystem1 ==
  Bus Selector : BusSelector  OutputSignals=V_PV,I_PV,I_diode,Irradiance (W/m2),Temperature (deg C)
  Demux : Demux  Outputs=2
  Gain : Gain  Gain=-1
  IdIq (pu) VSC Control : Scope  NumInputPorts=2
  MPPT Algorithm : Scope
  Mux : Mux  Inputs=2
  Mux2 : Mux  Inputs=2
  PV : Scope  NumInputPorts=3
  Power (Positive-Sequence) : spsPowerPositiveSequenceLib/Power (Positive-Sequence)  Freq=60  Vinit=[0, 0]  Iinit=[0, 0]  Ts=Ts_Control
  Selector : Selector  InputPortWidth=3  IndexOptions=Index vector (dialog)  Indices=[1]  OutputSizes=1
  Selector1 : Selector  InputPortWidth=3  IndexOptions=Index vector (dialog)  Indices=[1]  OutputSizes=1
  Terminator1 : Terminator
  W2kW : Gain  Gain=1/1000
  tag scope: I_PV=global, Ia_B1=global, Idiode_PV=global, Ir=global, P_B1_kW=global, Temp=global, V_PV=global, Va_B1=global
  wires:
  [Vabc_B1] -> Power (Positive-Sequence)/1, Selector/1
  [Iabc_B1] -> Power (Positive-Sequence)/2, Selector1/1
  Power (Positive-Sequence)/1 -> W2kW/1
  [I_V_MPPT] -> Gain/1  "I_V"
  [IdIq_prim] -> Demux/1
  [Id_ref] -> Mux/1
  Demux/1 -> Mux/2
  Mux/1 -> IdIq (pu) VSC Control/1  "Idref Id (magenta)"
  Demux/2 -> IdIq (pu) VSC Control/2  "Iq"
  Selector/1 -> [Va_B1]
  Selector1/1 -> [Ia_B1]
  [V_PV] -> PV/1  "V_PV"
  [I_PV] -> PV/2  "I_PV"
  [Idiode_PV] -> PV/3  "Idiode_PV"
  [dI_dV_MPPT] -> Mux2/1  "dI/dV"
  Gain/1 -> Mux2/2  "-I/V"
  Mux2/1 -> MPPT Algorithm/1  "dI/dV     -I/V (magenta)"
  W2kW/1 -> [P_B1_kW]
  [m_PV] -> Bus Selector/1
  Bus Selector/1 -> [V_PV]  "<V_PV>"
  Bus Selector/2 -> [I_PV]  "<I_PV>"
  Bus Selector/4 -> [Ir]  "<Irradiance (W/m2)>"
  Bus Selector/3 -> [Idiode_PV]  "<I_diode>"
  Bus Selector/5 -> [Temp]  "<Temperature (deg C)>"
  Power (Positive-Sequence)/2 -> Terminator1/1

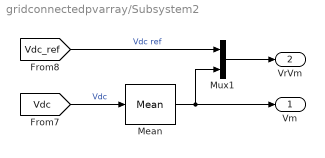
== system gridconnectedpvarray/Subsystem2 ==
  Mean : spsMeanLib/Mean  Freq=60  Vinit=0  Ts=Ts_Control
  Mux1 : Mux  Inputs=2
  Vm : Outport  VectorParamsAs1DForOutWhenUnconnected=off
  VrVm : Outport  Port=2  VectorParamsAs1DForOutWhenUnconnected=off
  wires:
  [Vdc_ref] -> Mux1/1  "Vdc ref"
  [Vdc] -> Mean/1  "Vdc"
  Mux1/1 -> VrVm/1
  Mean/1 -> Mux1/2, Vm/1

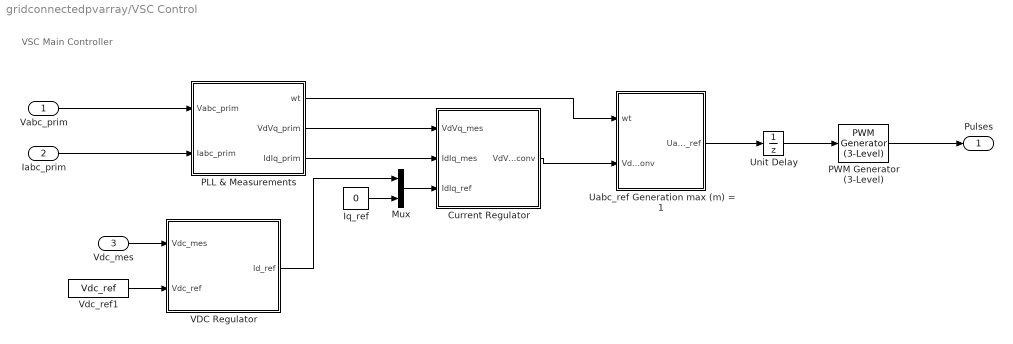
== system gridconnectedpvarray/VSC Control ==
  note: VSC Main Controller
  Vabc_prim : Inport  PortDimensions=3
  Iabc_prim : Inport  Port=2  PortDimensions=3
  Vdc_mes : Inport  Port=3  PortDimensions=1
  Current Regulator : Subsystem
  Iq_ref : Constant  Value=0
  Mux : Mux  Inputs=2
  PLL & Measurements : Subsystem
  PWM Generator (3-Level) : spsPWMGenerator3LevelLib/PWM Generator (3-Level)  ModulatorType=Three-phase bridge (12 pulses)  ModulatorMode=Unsynchronized  nF=27  Fc=33*60  ModulatingSignals=off  m=0.8  Freq=60  Phase=0  Ts=Ts_Power
  Uabc_ref Generation max (m) = 1 : Subsystem
  Unit Delay : UnitDelay  SampleTime=Ts_Control  HasFrameUpgradeWarning=on
  VDC Regulator : Subsystem
  Vdc_ref1 : Constant  Value=Vdc_ref
  Pulses : Outport  VectorParamsAs1DForOutWhenUnconnected=off
  wires:
  VDC Regulator/1(Id_ref) -> Mux/1
  PLL & Measurements/1(wt) -> Uabc_ref Generation max (m) = 1/1(wt)
  Current Regulator/1(VdVq_conv) -> Uabc_ref Generation max (m) = 1/2(VdVq_conv)
  Iq_ref/1 -> Mux/2
  Mux/1 -> Current Regulator/3(IdIq_ref)
  PLL & Measurements/3(IdIq_prim) -> Current Regulator/2(IdIq_mes)
  PLL & Measurements/2(VdVq_prim) -> Current Regulator/1(VdVq_mes)
  Vdc_mes/1 -> VDC Regulator/1(Vdc_mes)
  Vabc_prim/1 -> PLL & Measurements/1(Vabc_prim)
  Iabc_prim/1 -> PLL & Measurements/2(Iabc_prim)
  Unit Delay/1 -> PWM Generator (3-Level)/1
  PWM Generator (3-Level)/1 -> Pulses/1
  Uabc_ref Generation max (m) = 1/1(Uabc_ref) -> Unit Delay/1
  Vdc_ref1/1 -> VDC Regulator/2(Vdc_ref)

== system gridconnectedpvarray/info ==

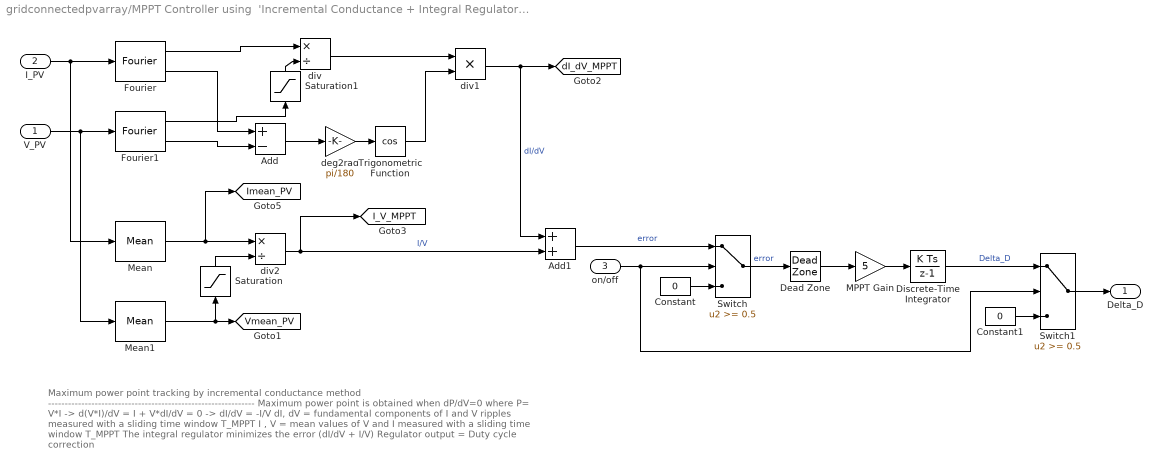
== system gridconnectedpvarray/MPPT Controller using  'Incremental Conductance + Integral Regulator'  technique /MPPT ==
  note: Maximum power point tracking by incremental conductance method
      | --------------------------------------------------------------
      | Maximum power point is obtained when dP/dV=0  where P= V*I
      | -> d(V*I)/dV = I + V*dI/dV = 0
      | -> dI/dV = -I/V
      |
      | dI, dV  = fundamental components of I and V ripples measured with a sliding time window T_MPPT
      | I , V   = mean values of V and I measured with a sliding time window T_MPPT
      |
      | The integral regulator minimizes the error (dI/dV + I/V)
      | Regulator output = Duty cycle correction
  V_PV : Inport
  I_PV : Inport  Port=2
  on/off : Inport  Port=3
  Add : Sum  Inputs=+-
  Add1 : Sum
  Constant : Constant  Value=0
  Constant1 : Constant  Value=0
  Dead Zone : DeadZone  LowerValue=-0.05  UpperValue=0.05
  Discrete-Time Integrator : DiscreteIntegrator  SampleTime=Ts_Control  LimitOutput=on  UpperSaturationLimit=1  LowerSaturationLimit=-1  ICPrevOutput=DiscIntNeverNeededParam  ICPrevScaledInput=DiscIntNeverNeededParam
  Fourier : spsFourierLib/Fourier  Freq=1/T_MPPT  n=1  InInit=[0, 0]  Ts=Ts_Control
  Fourier1 : spsFourierLib/Fourier  Freq=1/T_MPPT  n=1  InInit=[0, 0]  Ts=Ts_Control
  MPPT Gain : Gain  Gain=5
  Mean : spsMeanLib/Mean  Freq=1/T_MPPT  Vinit=0  Ts=Ts_Control
  Mean1 : spsMeanLib/Mean  Freq=1/T_MPPT  Vinit=0  Ts=Ts_Control
  Saturation : Saturate  UpperLimit=inf  LowerLimit=eps
  Saturation1 : Saturate  UpperLimit=inf  LowerLimit=eps
  Switch : Switch  Threshold=0.5  SaturateOnIntegerOverflow=off  InputSameDT=off
  Switch1 : Switch  Threshold=0.5  SaturateOnIntegerOverflow=off  InputSameDT=off
  Trigonometric Function : Trigonometry  Operator=cos
  deg2rad : Gain  Gain=pi/180
  div : Product  Inputs=*/  RndMeth=Zero
  div1 : Product  Inputs=**  RndMeth=Zero
  div2 : Product  Inputs=*/  RndMeth=Zero
  Delta_D : Outport  VectorParamsAs1DForOutWhenUnconnected=off
  tag scope: I_V_MPPT=global, Imean_PV=global, Vmean_PV=global, dI_dV_MPPT=global
  wires:
  Dead Zone/1 -> MPPT Gain/1
  Switch/1 -> Dead Zone/1  "error"
  Saturation1/1 -> div/2
  Saturation/1 -> div2/2
  Switch1/1 -> Delta_D/1
  on/off/1 -> Switch/2, Switch1/2
  Constant1/1 -> Switch1/3
  Discrete-Time Integrator/1 -> Switch1/1  "Delta_D"
  Constant/1 -> Switch/3
  MPPT Gain/1 -> Discrete-Time Integrator/1
  Add1/1 -> Switch/1  "error"
  div2/1 -> Add1/2, [I_V_MPPT]  "I/V"
  Mean1/1 -> Saturation/1, [Vmean_PV]
  Mean/1 -> div2/1, [Imean_PV]
  div1/1 -> Add1/1, [dI_dV_MPPT]  "dI/dV"
  Trigonometric Function/1 -> div1/2
  div/1 -> div1/1
  deg2rad/1 -> Trigonometric Function/1
  Add/1 -> deg2rad/1
  Fourier1/1 -> Saturation1/1
  Fourier1/2 -> Add/2
  Fourier/2 -> Add/1
  V_PV/1 -> Mean1/1, Fourier1/1
  I_PV/1 -> Mean/1, Fourier/1
  Fourier/1 -> div/1
